simulink model "sysp3_LA"  (R2023a)
settings: Solver=ode15s  StartTime=0.0  StopTime=10  MaxStep=1e-3  RelTol=1e-3
settings Model: Creator=miros  LastModifiedBy=miros
settings DataIOCC: ReturnWorkspaceOutputs=off  TimeSaveName=t
settings DebuggingCC: AlgebraicLoopMsg=none  ArtificialAlgebraicLoopMsg=none  BlockPriorityViolationMsg=error  MinStepSizeMsg=error  MaxConsecutiveZCsMsg=none  ModelReferenceExtraNoncontSigs=none  OperatingPointInterfaceChecksumMismatchMsg=none

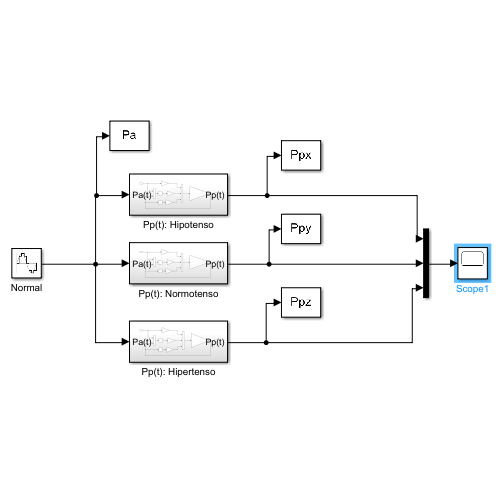
[thumbnail: Simulink's stored preview of the top-level diagram]
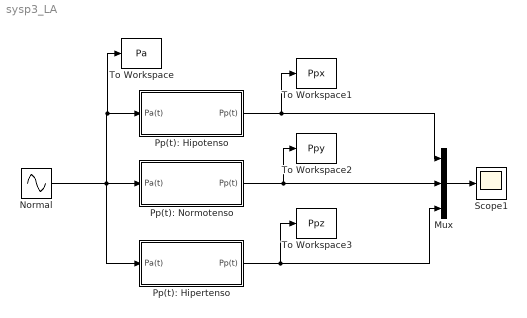
== system sysp3_LA ==
  Mux : Mux  Inputs=3
  Normal : Sin  Bias=0.8  Frequency=(2*pi)*(95/60)  SampleTime=0.001
  Pp(t): Hipertenso : Subsystem
  Pp(t): Hipotenso : Subsystem
  Pp(t): Normotenso : Subsystem
  Scope1 : Scope
  To Workspace : ToWorkspace  VariableName=Pa  SampleTime=-1
  To Workspace1 : ToWorkspace  VariableName=Ppx  SampleTime=-1
  To Workspace2 : ToWorkspace  VariableName=Ppy  SampleTime=-1
  To Workspace3 : ToWorkspace  VariableName=Ppz  SampleTime=-1
  wires:
  Mux/1 -> Scope1/1
  Normal/1 -> To Workspace/1, Pp(t): Hipotenso/1(Pa(t)), Pp(t): Normotenso/1(Pa(t)), Pp(t): Hipertenso/1(Pa(t))
  Pp(t): Hipotenso/1(Pp(t)) -> To Workspace1/1, Mux/1
  Pp(t): Normotenso/1(Pp(t)) -> To Workspace2/1, Mux/2
  Pp(t): Hipertenso/1(Pp(t)) -> To Workspace3/1, Mux/3

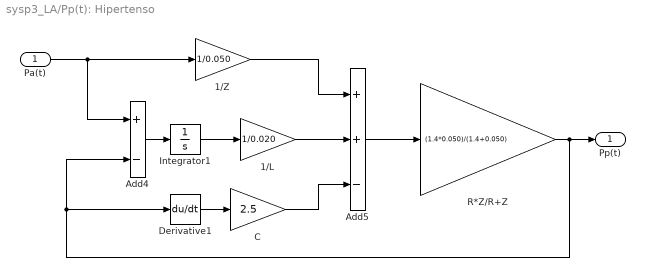
== system sysp3_LA/Pp(t): Hipertenso ==
  Pa(t) : Inport
  1/L : Gain  Gain=1/0.020
  1/Z : Gain  Gain=1/0.050
  Add4 : Sum  Inputs=+-
  Add5 : Sum  Inputs=++-
  C : Gain  Gain=2.5
  Derivative1 : Derivative
  Integrator1 : Integrator
  R*Z/R+Z : Gain  Gain=(1.4*0.050)/(1.4+0.050)
  Pp(t) : Outport  VectorParamsAs1DForOutWhenUnconnected=off
  wires:
  Add4/1 -> Integrator1/1
  Derivative1/1 -> C/1
  Integrator1/1 -> 1/L/1
  Pa(t)/1 -> Add4/1, 1/Z/1
  C/1 -> Add5/3
  Add5/1 -> R*Z/R+Z/1
  1/L/1 -> Add5/2
  R*Z/R+Z/1 -> Pp(t)/1, Derivative1/1, Add4/2
  1/Z/1 -> Add5/1

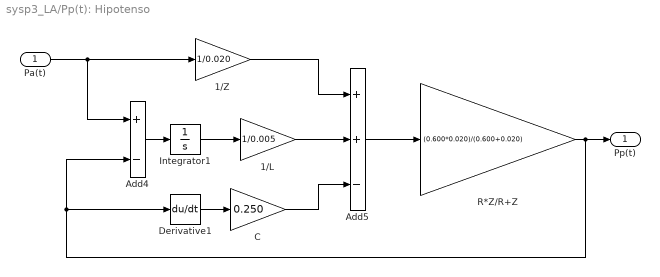
== system sysp3_LA/Pp(t): Hipotenso ==
  Pa(t) : Inport
  1/L : Gain  Gain=1/0.005
  1/Z : Gain  Gain=1/0.020
  Add4 : Sum  Inputs=+-
  Add5 : Sum  Inputs=++-
  C : Gain  Gain=0.250
  Derivative1 : Derivative
  Integrator1 : Integrator
  R*Z/R+Z : Gain  Gain=(0.600*0.020)/(0.600+0.020)
  Pp(t) : Outport  VectorParamsAs1DForOutWhenUnconnected=off
  wires:
  Add5/1 -> R*Z/R+Z/1
  Add4/1 -> Integrator1/1
  1/Z/1 -> Add5/1
  R*Z/R+Z/1 -> Pp(t)/1, Derivative1/1, Add4/2
  1/L/1 -> Add5/2
  Pa(t)/1 -> Add4/1, 1/Z/1
  Integrator1/1 -> 1/L/1
  Derivative1/1 -> C/1
  C/1 -> Add5/3

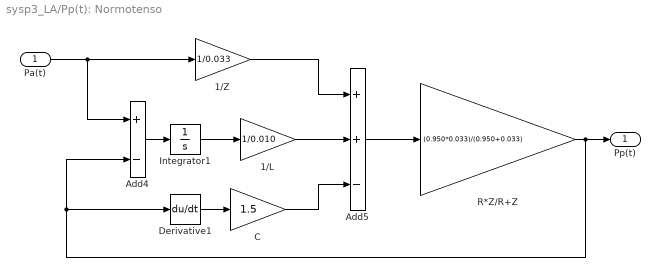
== system sysp3_LA/Pp(t): Normotenso ==
  Pa(t) : Inport
  1/L : Gain  Gain=1/0.010
  1/Z : Gain  Gain=1/0.033
  Add4 : Sum  Inputs=+-
  Add5 : Sum  Inputs=++-
  C : Gain  Gain=1.5
  Derivative1 : Derivative
  Integrator1 : Integrator
  R*Z/R+Z : Gain  Gain=(0.950*0.033)/(0.950+0.033)
  Pp(t) : Outport  VectorParamsAs1DForOutWhenUnconnected=off
  wires:
  Integrator1/1 -> 1/L/1
  Pa(t)/1 -> Add4/1, 1/Z/1
  R*Z/R+Z/1 -> Pp(t)/1, Derivative1/1, Add4/2
  1/Z/1 -> Add5/1
  1/L/1 -> Add5/2
  Add5/1 -> R*Z/R+Z/1
  C/1 -> Add5/3
  Add4/1 -> Integrator1/1
  Derivative1/1 -> C/1
